simulink model "sampleModel1518"  (R2023a)
settings: Solver=VariableStepAuto  StartTime=0.0  StopTime=10.0  RelTol=1e-3
libraries: hdlsllib x5, simulink x1
settings Model: Creator=user1  LastModifiedBy=user1

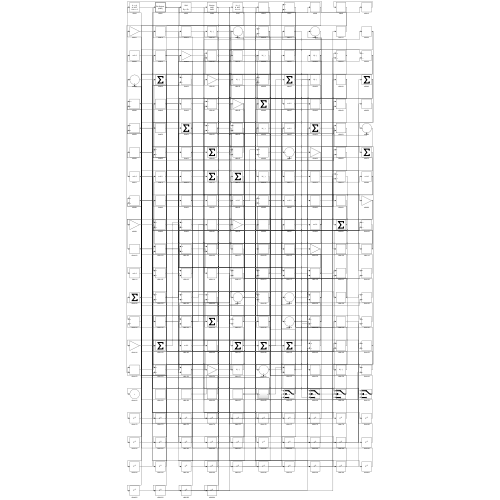
[thumbnail: Simulink's stored preview of the top-level diagram]
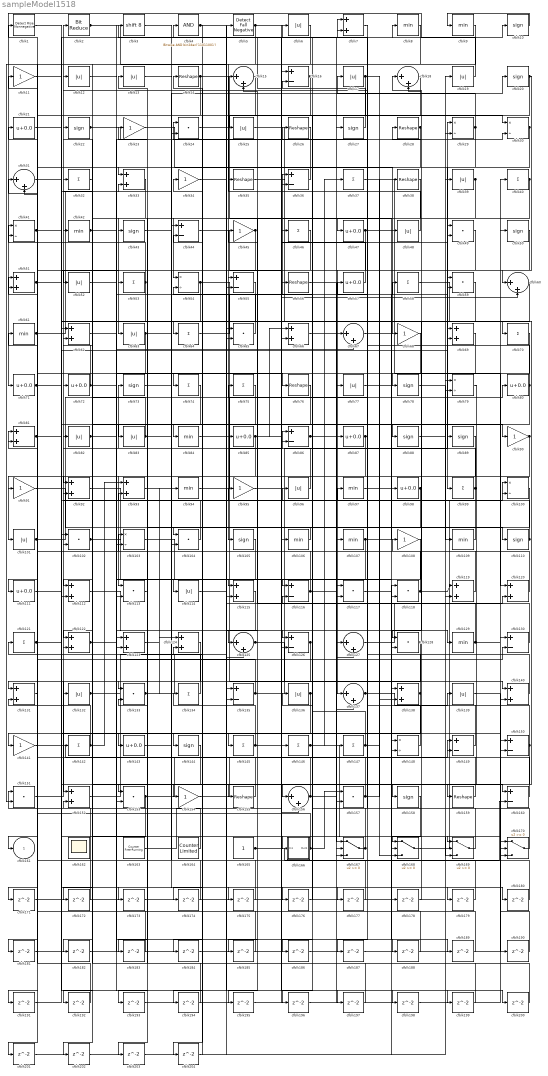
== system sampleModel1518 ==
  cfblk1 : hdlsllib/Logic and Bit Operations/Detect Rise Nonnegative  vinit=0  OutDataTypeStr=boolean
  cfblk{10,20,22,27,43,50,73,78,88..89,105,110,144,158} (14 alike) : Signum
  cfblk{29..30,41,54,79,100,103,148} (8 alike) : Product  Inputs=*/  RndMeth=Zero  SaturateOnIntegerOverflow=on
  cfblk{6,12..13,17,19,25,39,48,52,63,77,82..83,96,101,114,132,136,139} (19 alike) : Abs  SaturateOnIntegerOverflow=off
  cfblk{24,49,59,65,102,104,113,117..118,128,133,151,153,157} (14 alike) : DotProduct  OutDataTypeStr=Inherit: Inherit via internal rule
  cfblk{8..9,42,61,84,94,97,106..107,109,129} (11 alike) : MinMax
  cfblk{11,23,34,45,68,90..91,95,108,141,154} (11 alike) : Gain
  cfblk{21,47,57,71..72,80,85,87,98,111,143} (11 alike) : Bias  Bias=0.0  SaturateOnIntegerOverflow=off
  cfblk{7,33,51,62,66,69,81,92..93,112,115,119..120,122..124,131,138,140,152} (20 alike) : Sum
  cfblk{16,36,44,55,86,116,126,130,135,149..150,160} (12 alike) : Sum  Inputs=+-
  cfblk{32,37,40,46,53,58,64,70,74..75,99,121,134,142,145..147} (17 alike) : Sum  Inputs=+
  cfblk{15,18,31,60,67,125,127,137,156} (9 alike) : Sum  Inputs=|++
  cfblk{14,26,28,35,38,56,76,155,159} (9 alike) : Reshape
  cfblk162 : Scope
      settings: Floating=on
  cfblk163 : hdlsllib/Sources/Counter Free-Running  NumBits=16  tsamp=-1
  cfblk164 : hdlsllib/Sources/Counter Limited  uplimit=7  tsamp=-1
  cfblk165 : Constant  SampleTime=-1
  cfblk166 : Subsystem
      settings: LibrarySourceBlock=|
      | hdlsllib/Ports &
      | Subsystems/Subsystem
  cfblk{167..170} (4 alike) : Switch  SaturateOnIntegerOverflow=off  InputSameDT=off
  cfblk{171..204} (34 alike) : Delay  SampleTime=1
  cfblk2 : hdlsllib/Logic and Bit Operations/Bit Reduce  mode=AND
  cfblk3 : ArithShift  BitShiftNumber=8
  cfblk4 : simulink/Logic and Bit Operations/Bitwise Operator  logicop=AND  UseBitMask=on  BitMask=bin2dec('11011001')  BitMaskRealWorld=Stored Integer
      settings: LibrarySourceBlock=|
      | hdlsllib/Logic and Bit
      | Operations/Bitwise
      | Operator
  cfblk5 : hdlsllib/Logic and Bit Operations/Detect Fall Negative  vinit=0  OutDataTypeStr=boolean
  cfblk161 : Outport  VectorParamsAs1DForOutWhenUnconnected=off
  wires:
  cfblk104/1 -> cfblk2/1
  cfblk151/1 -> cfblk72/1
  cfblk85/1 -> cfblk66/1, cfblk168/2, cfblk184/1
  cfblk80/1 -> cfblk6/1, cfblk112/1, cfblk128/1
  cfblk89/1 -> cfblk101/1
  cfblk25/1 -> cfblk137/1
  cfblk10/1 -> cfblk9/1
  cfblk58/1 -> cfblk151/1
  cfblk27/1 -> cfblk4/1
  cfblk39/1 -> cfblk63/1, cfblk195/1
  cfblk69/1 -> cfblk78/1
  cfblk157/1 -> cfblk32/1, cfblk48/1
  cfblk50/1 -> cfblk67/1
  cfblk87/1 -> cfblk113/1, cfblk57/1
  cfblk56/1 -> cfblk107/1
  cfblk120/1 -> cfblk26/1
  cfblk14/1 -> cfblk47/1, cfblk52/1
  cfblk84/1 -> cfblk86/1
  cfblk138/1 -> cfblk18/1, cfblk93/2, cfblk201/1
  cfblk129/1 -> cfblk50/1, cfblk15/2, cfblk95/1
  cfblk30/1 -> cfblk99/1, cfblk191/1
  cfblk99/1 -> cfblk73/1, cfblk92/2
  cfblk101/1 -> cfblk80/1, cfblk200/1
  cfblk19/1 -> cfblk71/1
  cfblk168/1 -> cfblk40/1
  cfblk54/1 -> cfblk140/1, cfblk112/2
  cfblk159/1 -> cfblk97/1
  cfblk29/1 -> cfblk105/1, cfblk17/1
  cfblk5/1 -> cfblk55/1, cfblk198/1
  cfblk40/1 -> cfblk43/1, cfblk153/1
  cfblk37/1 -> cfblk120/1
  cfblk153/1 -> cfblk149/1, cfblk192/1
  cfblk60/1 -> cfblk88/1
  cfblk140/1 -> cfblk75/1
  cfblk44/1 -> cfblk146/1
  cfblk24/1 -> cfblk30/1
  cfblk125/1 -> cfblk29/1, cfblk147/1
  cfblk38/1 -> cfblk54/1
  cfblk42/1 -> cfblk74/1, cfblk154/1
  cfblk32/1 -> cfblk92/1
  cfblk148/1 -> cfblk12/1
  cfblk9/1 -> cfblk151/2
  cfblk62/1 -> cfblk160/1
  cfblk105/1 -> cfblk123/2
  cfblk1/1 -> cfblk53/1
  cfblk31/1 -> cfblk70/1
  cfblk146/1 -> cfblk169/1, cfblk37/1
  cfblk64/1 -> cfblk36/1
  cfblk155/1 -> cfblk82/1
  cfblk97/1 -> cfblk98/1
  cfblk131/1 -> cfblk51/1
  cfblk86/1 -> cfblk127/2, cfblk69/1
  cfblk119/1 -> cfblk41/1
  cfblk109/1 -> cfblk56/1
  cfblk17/1 -> cfblk161/1, cfblk168/3
  cfblk165/1 -> cfblk160/2, cfblk60/2
  cfblk72/1 -> cfblk110/1, cfblk42/1
  cfblk150/1 -> cfblk102/2, cfblk157/2
  cfblk123/1 -> cfblk124/1
  cfblk124/1 -> cfblk152/1
  cfblk141/1 -> cfblk149/2
  cfblk132/1 -> cfblk5/1, cfblk199/1
  cfblk57/1 -> cfblk46/1
  cfblk152/1 -> cfblk130/2
  cfblk170/1 -> cfblk7/1
  cfblk22/1 -> cfblk30/2, cfblk117/2
  cfblk158/1 -> cfblk168/1
  cfblk47/1 -> cfblk145/1, cfblk38/1
  cfblk137/1 -> cfblk139/1, cfblk189/1
  cfblk113/1 -> cfblk13/1
  cfblk66/1 -> cfblk87/1
  cfblk52/1 -> cfblk67/2
  cfblk82/1 -> cfblk25/1, cfblk188/1
  cfblk108/1 -> cfblk156/1
  cfblk142/1 -> cfblk51/2, cfblk93/1
  cfblk94/1 -> cfblk27/1
  cfblk112/1 -> cfblk137/2
  cfblk115/1 -> cfblk135/2
  cfblk126/1 -> cfblk131/1, cfblk143/1
  cfblk65/1 -> cfblk44/2
  cfblk48/1 -> cfblk15/1
  cfblk3/1 -> cfblk89/1
  cfblk35/1 -> cfblk118/2
  cfblk55/1 -> cfblk83/1
  cfblk28/1 -> cfblk77/1, cfblk202/1
  cfblk78/1 -> cfblk109/1
  cfblk169/1 -> cfblk54/2
  cfblk110/1 -> cfblk34/1, cfblk23/1
  cfblk164/1 -> cfblk61/1
  cfblk135/1 -> cfblk79/1, cfblk21/1
  cfblk13/1 -> cfblk76/1
  cfblk136/1 -> cfblk16/2, cfblk172/1
  cfblk98/1 -> cfblk28/1, cfblk203/1
  cfblk8/1 -> cfblk141/1
  cfblk134/1 -> cfblk121/1
  cfblk96/1 -> cfblk22/1
  cfblk6/1 -> cfblk132/1
  cfblk81/1 -> cfblk10/1, cfblk69/2, cfblk153/2
  cfblk15/1 -> cfblk55/2
  cfblk33/1 -> cfblk122/1
  cfblk92/1 -> cfblk156/2
  cfblk12/1 -> cfblk115/1
  cfblk26/1 -> cfblk111/1
  cfblk116/1 -> cfblk45/1, cfblk8/1
  cfblk91/1 -> cfblk167/1
  cfblk70/1 -> cfblk125/1
  cfblk76/1 -> cfblk144/1
  cfblk18/1 -> cfblk116/1
  cfblk149/1 -> cfblk24/1
  cfblk74/1 -> cfblk113/2
  cfblk23/1 -> cfblk68/1
  cfblk71/1 -> cfblk166/1(In1), cfblk158/1
  cfblk83/1 -> cfblk62/2, cfblk179/1
  cfblk156/1 -> cfblk103/1, cfblk49/2
  cfblk41/1 -> cfblk150/2, cfblk171/1
  cfblk160/1 -> cfblk81/1
  cfblk121/1 -> cfblk81/2, cfblk100/2
  cfblk88/1 -> cfblk39/1
  cfblk2/1 -> cfblk85/1, cfblk128/2
  cfblk75/1 -> cfblk133/1
  cfblk53/1 -> cfblk11/1, cfblk103/2
  cfblk127/1 -> cfblk19/1
  cfblk43/1 -> cfblk90/1
  cfblk11/1 -> cfblk84/1
  cfblk133/1 -> cfblk120/2, cfblk94/1
  cfblk147/1 -> cfblk96/1, cfblk138/2
  cfblk73/1 -> cfblk170/2
  cfblk154/1 -> cfblk106/1
  cfblk95/1 -> cfblk7/2
  cfblk122/1 -> cfblk59/1, cfblk126/1
  cfblk103/1 -> cfblk117/1
  cfblk145/1 -> cfblk49/1, cfblk134/1
  cfblk90/1 -> cfblk185/1, cfblk186/1
  cfblk77/1 -> cfblk138/1
  cfblk167/1 -> cfblk136/1, cfblk3/1
  cfblk102/1 -> cfblk148/1, cfblk58/1
  cfblk61/1 -> cfblk24/2, cfblk33/2
  cfblk63/1 -> cfblk142/1, cfblk129/1
  cfblk79/1 -> cfblk159/1
  cfblk130/1 -> cfblk35/1
  cfblk163/1 -> cfblk100/1
  cfblk117/1 -> cfblk170/3
  cfblk20/1 -> cfblk60/1, cfblk196/1
  cfblk45/1 -> cfblk91/1, cfblk104/2
  cfblk16/1 -> cfblk65/2, cfblk114/1
  cfblk143/1 -> cfblk20/1
  cfblk128/1 -> cfblk108/1, cfblk193/1
  cfblk4/1 -> cfblk64/1, cfblk66/2
  cfblk51/1 -> cfblk175/1, cfblk176/1
  cfblk36/1 -> cfblk33/1
  cfblk107/1 -> cfblk59/2, cfblk194/1
  cfblk106/1 -> cfblk104/1
  cfblk166/1(Out1) -> cfblk31/1, cfblk157/1, cfblk122/2
  cfblk21/1 -> cfblk169/3
  cfblk49/1 -> cfblk155/1
  cfblk118/1 -> cfblk119/1, cfblk36/2
  cfblk171/1 -> cfblk29/2
  cfblk172/1 -> cfblk41/2
  cfblk111/1 -> cfblk173/1
  cfblk173/1 -> cfblk127/1
  cfblk59/1 -> cfblk174/1
  cfblk174/1 -> cfblk44/1
  cfblk175/1 -> cfblk131/2
  cfblk176/1 -> cfblk116/2
  cfblk93/1 -> cfblk177/1
  cfblk177/1 -> cfblk16/1
  cfblk67/1 -> cfblk178/1
  cfblk178/1 -> cfblk18/2
  cfblk179/1 -> cfblk169/2
  cfblk34/1 -> cfblk180/1
  cfblk180/1 -> cfblk65/1
  cfblk68/1 -> cfblk181/1
  cfblk181/1 -> cfblk86/2
  cfblk144/1 -> cfblk182/1
  cfblk182/1 -> cfblk123/1
  cfblk46/1 -> cfblk183/1
  cfblk183/1 -> cfblk102/1
  cfblk184/1 -> cfblk125/2
  cfblk185/1 -> cfblk1/1
  cfblk186/1 -> cfblk140/2
  cfblk7/1 -> cfblk187/1
  cfblk187/1 -> cfblk170/1
  cfblk188/1 -> cfblk135/1
  cfblk189/1 -> cfblk118/1
  cfblk139/1 -> cfblk190/1
  cfblk190/1 -> cfblk130/1
  cfblk191/1 -> cfblk62/1
  cfblk192/1 -> cfblk31/2
  cfblk193/1 -> cfblk167/3
  cfblk194/1 -> cfblk133/2
  cfblk195/1 -> cfblk126/2
  cfblk196/1 -> cfblk150/1
  cfblk114/1 -> cfblk197/1
  cfblk197/1 -> cfblk152/2
  cfblk198/1 -> cfblk119/2
  cfblk199/1 -> cfblk167/2
  cfblk200/1 -> cfblk124/2
  cfblk201/1 -> cfblk115/2
  cfblk202/1 -> cfblk79/2
  cfblk203/1 -> cfblk148/2
  cfblk100/1 -> cfblk204/1
  cfblk204/1 -> cfblk14/1

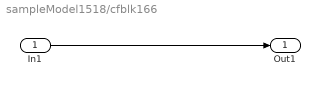
== system sampleModel1518/cfblk166 ==
  In1 : Inport
  Out1 : Outport
  wires:
  In1/1 -> Out1/1
